simulink model "EvPowertrainController"  (R2019b)
settings: Solver=ode4  StartTime=0.0  StopTime=inf  FixedStep=.01  RelTol=1e-3  EnableMultiTasking=on
model workspace (MAT data in the model file):
  BattChrgMax = -80000
  BattDischrgMax = 80000
  BrkPrsMax = 5000000
  ChrgLmt_bpt = [1 1 1 1 1 1 1 1 0.7 0.35 0]
  DischrgLmt_bpt = [0 0.35 0.7 1 1 1 1 1 1 1 1]
  MotMapEff = 0
  MotSpd = [0 1000 2000 2728.370453 3000 4000 5000 6000 7000 8000 9000 10000]
  MotTrq = [280 280 280 280 254.6479089 190.9859317 152.7887454 127.3239545 109.1348181 95.49296586 84.88263632 76.39437268]
  Ndiff = 7.94
  RegenBrkCutOff = [0 1]
  RegenBrkSpd_bpt = [5 9]
  Rm = 0.15
  SOC_bpt = [0 10 20 30 40 50 60 70 80 90 100]
  T_eff_bp = [0 20 40 60 80 100 120 140 160 180 200 220 240 260 280]
  disk_abore = 0.05
  efficiency_table = [85  85  85  85  85  85  85  85  85  85  85  85  85  85  85; 85  85  85  85  85  85  85  85  85  85  85  85  85  85  85; 85  85  90  90  90  90  90  90  90  90  88  88  88  88  88; 85  85  92  92  92  92  92  92  92  92  92  90  90  90  90; 85  85  92  92  93  93  93  93  92  92  92  90  90  90  90; 85  85  93  94  94  94  94  94  94  94  94  94  94  94  94; 85  85  93  94  94  95  95  95  95  95  95  95  95  95  95; 85  85  93  94  94  95  95  95  95  95  95  95  95  95  95; 85  85  93  94  95  95  95  95  95  95  95  95  95  95  95; 85  85  93  94  95  95  95  95  95  95  95  95  95  95  95; 85  85  93  94  94  94  94  94  94  94  94  94  94  94  94; 85  85  90  92  93  93  93  93  93  93  93  93  93  93  93]
  mu_kinetic = 0.35
  num_pads = 2
  w_eff_bp = [0 1000 2000 2728.370453 3000 4000 5000 6000 7000 8000 9000 10000]
libraries: simulink x6, autolibutils x1
settings Model: ModifiedByFormat=The MathWorks, Inc.  Creator=The MathWorks, Inc.  LastModifiedBy=The MathWorks, Inc.
settings DataIOCC: ReturnWorkspaceOutputs=off
settings DebuggingCC: UnderspecifiedInitializationDetection=Classic  MergeDetectMultiDrivingBlocksExec=none  SFNoUnconditionalDefaultTransitionDiag=warning  ArithmeticOperatorsInVariantConditions=warning
settings SFSimCC: SimUseLocalCustomCode=off  CustomCodeUndefinedFunction=UseInterfaceOnly
settings RTWCC: RTWUseLocalCustomCode=off
settings CodeAppCC: StateflowObjectComments=on
settings GRTTargetCC: TargetLangStandard=C89/C90 (ANSI)
settings ConfigComp: CovMetricSettings=dsw  CovHtmlReporting=on  CovSaveCumulativeToWorkspaceVar=on  CovSaveSingleToWorkspaceVar=on  CovShowResultsExplorer=off  CovExternalEMLEnable=off

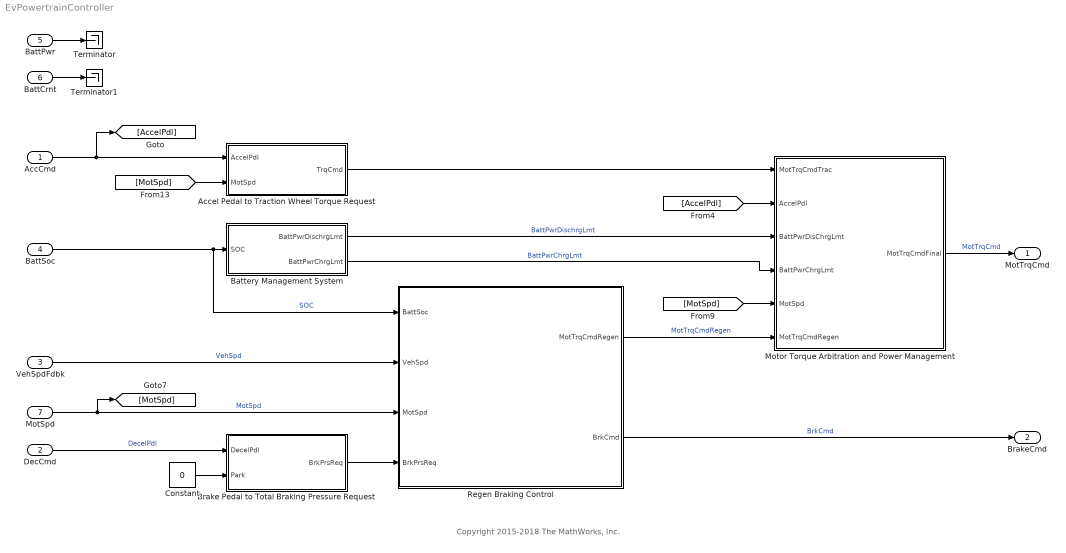
== system EvPowertrainController ==
  note: Copyright 2015-2018 The MathWorks, Inc.
  AccCmd : Inport
  DecCmd : Inport  Port=2  OutDataTypeStr=double
  VehSpdFdbk : Inport  Port=3
  BattSoc : Inport  Port=4
  BattPwr : Inport  Port=5
  BattCrnt : Inport  Port=6
  MotSpd : Inport  Port=7
  Accel Pedal to Traction Wheel Torque Request : Subsystem
  Battery Management System : Subsystem
  Brake Pedal to Total Braking Pressure Request : Subsystem
  Constant : Constant  Value=0
  Motor Torque Arbitration and Power Management : Subsystem
  Regen Braking Control : Subsystem  VariantControlMode=Label  Variant=on  VariantControl=(default)  LabelModeActiveChoice=Variant
  Terminator : Terminator
  Terminator1 : Terminator
  MotTrqCmd : Outport  VectorParamsAs1DForOutWhenUnconnected=off
  BrakeCmd : Outport  Port=2  VectorParamsAs1DForOutWhenUnconnected=off
  wires:
  [AccelPdl] -> Motor Torque Arbitration and Power Management/2(AccelPdl)
  Battery Management System/1(BattPwrDischrgLmt) -> Motor Torque Arbitration and Power Management/3(BattPwrDisChrgLmt)  "BattPwrDischrgLmt"
  DecCmd/1 -> Brake Pedal to Total Braking Pressure Request/1(DecelPdl)  "DecelPdl"
  Regen Braking Control/2(" BrkCmd") -> BrakeCmd/1  "BrkCmd"
  Constant/1 -> Brake Pedal to Total Braking Pressure Request/2(Park)
  Battery Management System/2(BattPwrChrgLmt) -> Motor Torque Arbitration and Power Management/4("BattPwrChrgLmt ")  "BattPwrChrgLmt"
  Brake Pedal to Total Braking Pressure Request/1(BrkPrsReq) -> Regen Braking Control/4("BrkPrsReq ")
  [MotSpd] -> Accel Pedal to Traction Wheel Torque Request/2(MotSpd)
  VehSpdFdbk/1 -> Regen Braking Control/2("VehSpd ")  "VehSpd"
  BattSoc/1 -> Regen Braking Control/1("BattSoc "), Battery Management System/1(SOC)  "SOC"
  Accel Pedal to Traction Wheel Torque Request/1(TrqCmd) -> Motor Torque Arbitration and Power Management/1(MotTrqCmdTrac)
  MotSpd/1 -> Regen Braking Control/3("MotSpd "), [MotSpd]  "MotSpd"
  AccCmd/1 -> [AccelPdl], Accel Pedal to Traction Wheel Torque Request/1(AccelPdl)
  [MotSpd] -> Motor Torque Arbitration and Power Management/5(MotSpd)
  Motor Torque Arbitration and Power Management/1(MotTrqCmdFinal) -> MotTrqCmd/1  "MotTrqCmd"
  Regen Braking Control/1(" MotTrqCmdRegen") -> Motor Torque Arbitration and Power Management/6(MotTrqCmdRegen)  "MotTrqCmdRegen"
  BattPwr/1 -> Terminator/1
  BattCrnt/1 -> Terminator1/1

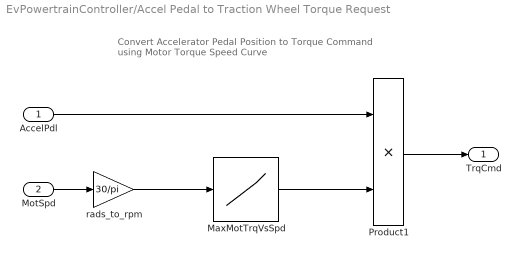
== system EvPowertrainController/Accel Pedal to Traction Wheel Torque Request ==
  note: Convert Accelerator Pedal Position to Torque Command
      | using Motor Torque Speed Curve
  AccelPdl : Inport
  MotSpd : Inport  Port=2
  MaxMotTrqVsSpd : Lookup_n-D  NumberOfTableDimensions=1  BreakpointsForDimension1=MotSpd  Table=MotTrq  ExtrapMethod=Clip  UseLastTableValue=on  InternalRulePriority=Speed  OutDataTypeStr=Inherit: Inherit from 'Table data'  RndMeth=Simplest  InputSameDT=on
  Product1 : Product
  rads_to_rpm : Gain  Gain=30/pi
  TrqCmd : Outport  VectorParamsAs1DForOutWhenUnconnected=off
  wires:
  Product1/1 -> TrqCmd/1
  MaxMotTrqVsSpd/1 -> Product1/2
  AccelPdl/1 -> Product1/1
  MotSpd/1 -> rads_to_rpm/1
  rads_to_rpm/1 -> MaxMotTrqVsSpd/1

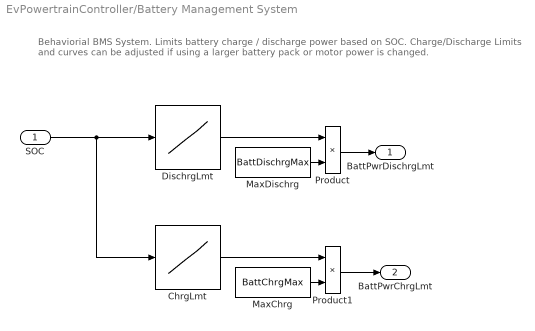
== system EvPowertrainController/Battery Management System ==
  note: Behaviorial BMS System. Limits battery charge / discharge power based on SOC.
      |
      | Charge/Discharge Limits and curves can be adjusted if using a larger battery pack
      | or motor power is changed.
  SOC : Inport
  ChrgLmt : Lookup_n-D  NumberOfTableDimensions=1  BreakpointsForDimension1=SOC_bpt  Table=ChrgLmt_bpt  ExtrapMethod=Clip  UseLastTableValue=on  InternalRulePriority=Speed  RndMeth=Simplest  InputSameDT=on
  DischrgLmt : Lookup_n-D  NumberOfTableDimensions=1  BreakpointsForDimension1=SOC_bpt  Table=DischrgLmt_bpt  ExtrapMethod=Clip  UseLastTableValue=on  InternalRulePriority=Speed  RndMeth=Simplest  InputSameDT=on
  MaxChrg : Constant  Value=BattChrgMax
  MaxDischrg : Constant  Value=BattDischrgMax
  Product : Product
  Product1 : Product
  BattPwrDischrgLmt : Outport  VectorParamsAs1DForOutWhenUnconnected=off
  BattPwrChrgLmt : Outport  Port=2  VectorParamsAs1DForOutWhenUnconnected=off
  wires:
  SOC/1 -> DischrgLmt/1, ChrgLmt/1
  MaxChrg/1 -> Product1/2
  MaxDischrg/1 -> Product/2
  Product/1 -> BattPwrDischrgLmt/1
  Product1/1 -> BattPwrChrgLmt/1
  ChrgLmt/1 -> Product1/1
  DischrgLmt/1 -> Product/1

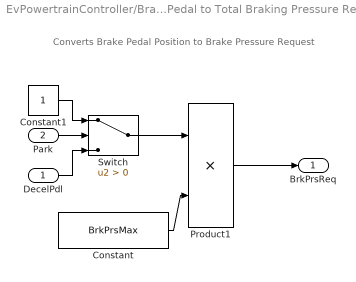
== system EvPowertrainController/Brake Pedal to Total Braking Pressure Request ==
  note: Converts Brake Pedal Position to Brake Pressure Request
  DecelPdl : Inport
  Park : Inport  Port=2
  Constant : Constant  Value=BrkPrsMax
  Constant1 : Constant
  Product1 : Product
  Switch : Switch  Criteria=u2 > Threshold
  BrkPrsReq : Outport  VectorParamsAs1DForOutWhenUnconnected=off
  wires:
  Constant/1 -> Product1/2
  Switch/1 -> Product1/1
  DecelPdl/1 -> Switch/3
  Constant1/1 -> Switch/1
  Product1/1 -> BrkPrsReq/1
  Park/1 -> Switch/2

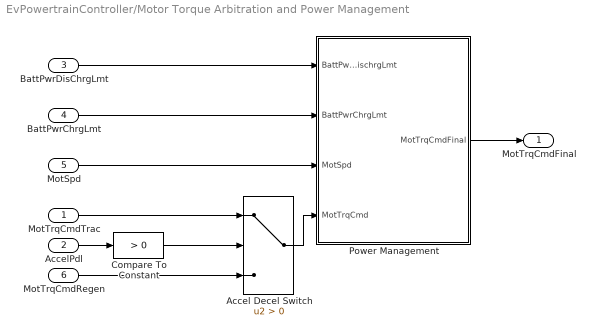
== system EvPowertrainController/Motor Torque Arbitration and Power Management ==
  MotTrqCmdTrac : Inport
  AccelPdl : Inport  Port=2
  BattPwrDisChrgLmt : Inport  Port=3
  "BattPwrChrgLmt " : Inport  Port=4
  MotSpd : Inport  Port=5
  MotTrqCmdRegen : Inport  Port=6
  Accel Decel Switch : Switch  Criteria=u2 > Threshold
  Compare To Constant : simulink/Logic and Bit Operations/Compare To Constant  relop=>  const=0  OutDataTypeStr=boolean
  Power Management : Subsystem
  MotTrqCmdFinal : Outport  VectorParamsAs1DForOutWhenUnconnected=off
  wires:
  AccelPdl/1 -> Compare To Constant/1
  MotTrqCmdRegen/1 -> Accel Decel Switch/3
  MotTrqCmdTrac/1 -> Accel Decel Switch/1
  Power Management/1(MotTrqCmdFinal) -> MotTrqCmdFinal/1
  Accel Decel Switch/1 -> Power Management/4(MotTrqCmd)
  BattPwrDisChrgLmt/1 -> Power Management/1(BattPwrDischrgLmt)
  "BattPwrChrgLmt "/1 -> Power Management/2(BattPwrChrgLmt)
  MotSpd/1 -> Power Management/3(MotSpd)
  Compare To Constant/1 -> Accel Decel Switch/2

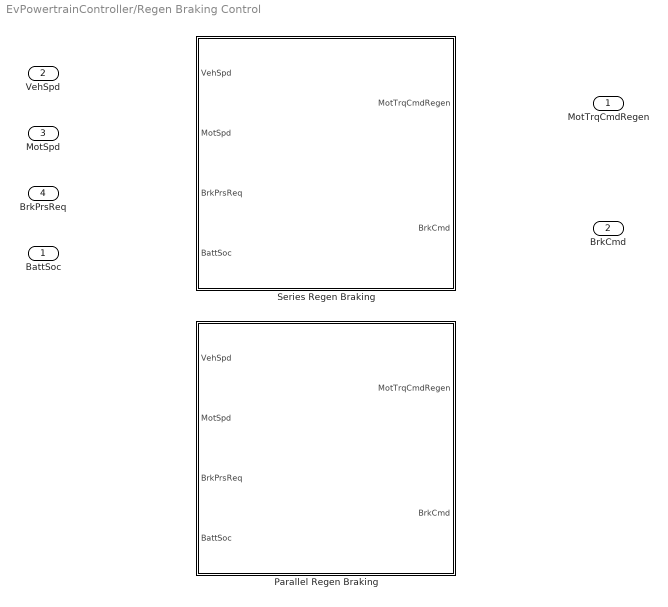
== system EvPowertrainController/Regen Braking Control ==
  "BattSoc " : Inport
  "VehSpd " : Inport  Port=2
  "MotSpd " : Inport  Port=3
  "BrkPrsReq " : Inport  Port=4
  Parallel Regen Braking : Subsystem  InitFcn=%[~]=autosharedicon('autolibutils',gcb,0);  VariantControl=(default)
  Series Regen Braking : Subsystem  InitFcn=%[~]=autosharedicon('autolibutils',gcb,0);  VariantControl=Variant
  " MotTrqCmdRegen" : Outport  VectorParamsAs1DForOutWhenUnconnected=off
  " BrkCmd" : Outport  Port=2  VectorParamsAs1DForOutWhenUnconnected=off

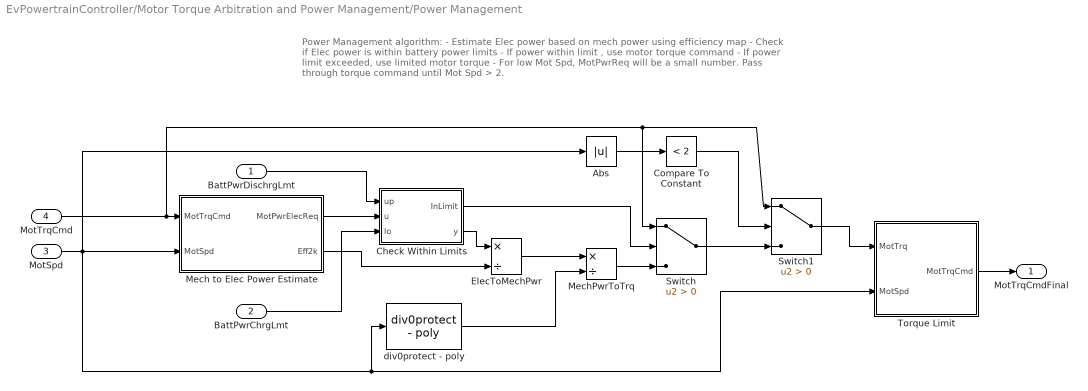
== system EvPowertrainController/Motor Torque Arbitration and Power Management/Power Management ==
  note: Power Management algorithm:
      | - Estimate Elec power based on mech power using efficiency map
      | - Check if Elec power is within battery power limits
      | - If power within limit , use motor torque command
      | - If power limit exceeded, use limited motor torque
      | - For low Mot Spd, MotPwrReq will be a small number.  Pass through torque command until Mot Spd > 2.
  BattPwrDischrgLmt : Inport
  BattPwrChrgLmt : Inport  Port=2
  MotSpd : Inport  Port=3
  MotTrqCmd : Inport  Port=4
  Abs : Abs
  Check Within Limits : Subsystem
  Compare To Constant : simulink/Logic and Bit Operations/Compare To Constant  relop=<  const=2  OutDataTypeStr=boolean
  ElecToMechPwr : Product  Inputs=*/
  Mech to Elec Power Estimate : Subsystem
  MechPwrToTrq : Product  Inputs=*/
  Switch : Switch  Criteria=u2 > Threshold
  Switch1 : Switch  Criteria=u2 > Threshold
  Torque Limit : Subsystem
  div0protect - poly : autolibutils/div0protect - poly  thresh=2  aMode=aMode
      settings: SourceProductName=Powertrain Blockset  SourceProductBaseCode=PW
  MotTrqCmdFinal : Outport  VectorParamsAs1DForOutWhenUnconnected=off
  wires:
  MotSpd/1 -> Abs/1, Torque Limit/2(MotSpd), div0protect - poly/1, Mech to Elec Power Estimate/2(MotSpd)
  MotTrqCmd/1 -> Switch/1, Switch1/1, Mech to Elec Power Estimate/1(MotTrqCmd)
  div0protect - poly/1 -> MechPwrToTrq/2
  Mech to Elec Power Estimate/2(Eff2k) -> ElecToMechPwr/2
  ElecToMechPwr/1 -> MechPwrToTrq/1
  MechPwrToTrq/1 -> Switch/3
  Torque Limit/1(MotTrqCmd) -> MotTrqCmdFinal/1
  BattPwrDischrgLmt/1 -> Check Within Limits/1(up)
  Mech to Elec Power Estimate/1(MotPwrElecReq) -> Check Within Limits/2(u)
  BattPwrChrgLmt/1 -> Check Within Limits/3(lo)
  Check Within Limits/2(y) -> ElecToMechPwr/1
  Switch/1 -> Switch1/3
  Check Within Limits/1(InLimit) -> Switch/2
  Switch1/1 -> Torque Limit/1(MotTrq)
  Abs/1 -> Compare To Constant/1
  Compare To Constant/1 -> Switch1/2

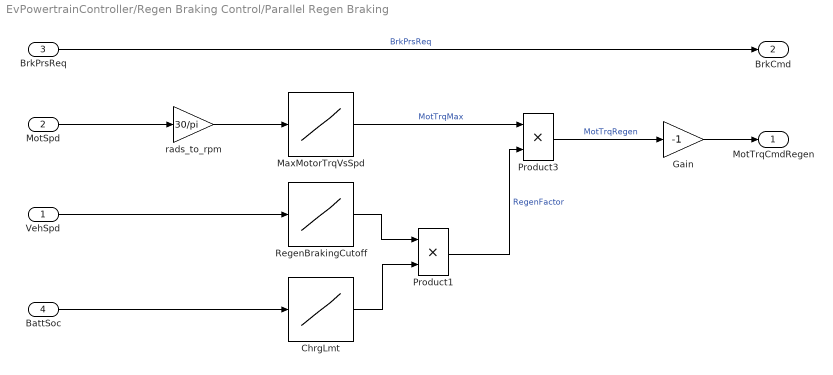
== system EvPowertrainController/Regen Braking Control/Parallel Regen Braking ==
  VehSpd : Inport
  MotSpd : Inport  Port=2
  "BrkPrsReq " : Inport  Port=3
  BattSoc : Inport  Port=4
  ChrgLmt : Lookup_n-D  NumberOfTableDimensions=1  BreakpointsForDimension1=[0:10:100]  Table=[1 1 1 1 1 1 1 1 0.7 0.35 0]  ExtrapMethod=Clip  UseLastTableValue=on  InternalRulePriority=Speed  RndMeth=Simplest  InputSameDT=on
  Gain : Gain  Gain=-1
  MaxMotorTrqVsSpd : Lookup_n-D  NumberOfTableDimensions=1  BreakpointsForDimension1=MotSpd  Table=MotTrq  ExtrapMethod=Clip  UseLastTableValue=on  InternalRulePriority=Speed  OutDataTypeStr=Inherit: Inherit from 'Table data'  RndMeth=Simplest  InputSameDT=on
  Product1 : Product
  Product3 : Product
  RegenBrakingCutoff : Lookup_n-D  NumberOfTableDimensions=1  BreakpointsForDimension1=[2.2 4.5]  Table=[0 1]  ExtrapMethod=Clip  UseLastTableValue=on  InternalRulePriority=Speed  RndMeth=Simplest  InputSameDT=on
  rads_to_rpm : Gain  Gain=30/pi
  " MotTrqCmdRegen" : Outport  VectorParamsAs1DForOutWhenUnconnected=off
  " BrkCmd" : Outport  Port=2  VectorParamsAs1DForOutWhenUnconnected=off
  wires:
  Gain/1 -> " MotTrqCmdRegen"/1
  BattSoc/1 -> ChrgLmt/1
  Product3/1 -> Gain/1  "MotTrqRegen"
  Product1/1 -> Product3/2  "RegenFactor"
  RegenBrakingCutoff/1 -> Product1/1
  VehSpd/1 -> RegenBrakingCutoff/1
  ChrgLmt/1 -> Product1/2
  MaxMotorTrqVsSpd/1 -> Product3/1  "MotTrqMax"
  rads_to_rpm/1 -> MaxMotorTrqVsSpd/1
  MotSpd/1 -> rads_to_rpm/1
  "BrkPrsReq "/1 -> " BrkCmd"/1  "BrkPrsReq"

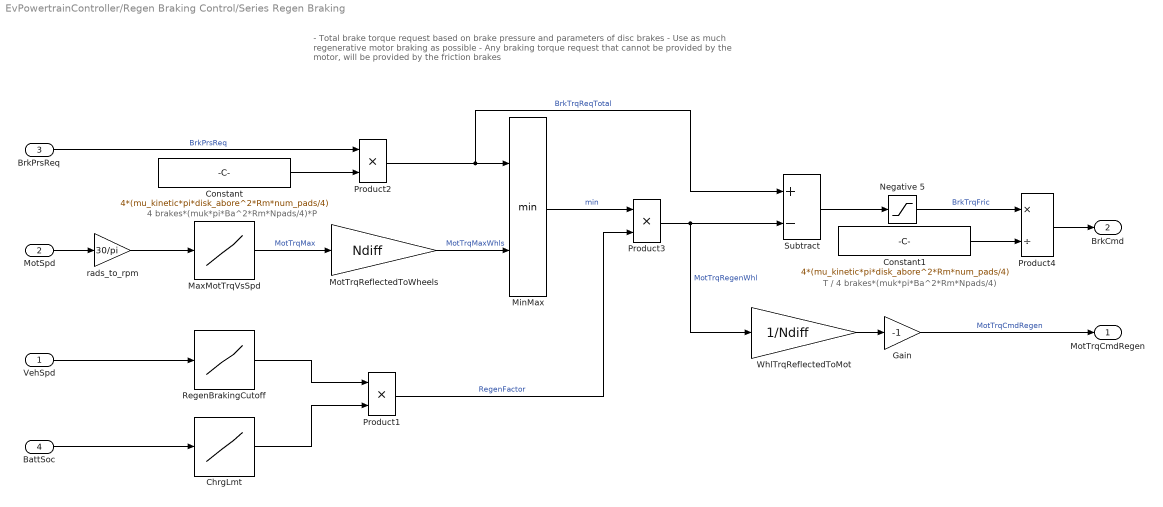
== system EvPowertrainController/Regen Braking Control/Series Regen Braking ==
  note: - Total brake torque request based on brake pressure and parameters of disc brakes
      | - Use as much regenerative motor braking as possible
      | - Any braking torque request that cannot be provided by the motor, will be provided by the friction brakes
  note: T / 4 brakes*(muk*pi*Ba^2*Rm*Npads/4)
  note: 4 brakes*(muk*pi*Ba^2*Rm*Npads/4)*P
  VehSpd : Inport
  MotSpd : Inport  Port=2
  "BrkPrsReq " : Inport  Port=3
  BattSoc : Inport  Port=4
  ChrgLmt : Lookup_n-D  NumberOfTableDimensions=1  BreakpointsForDimension1=SOC_bpt  Table=ChrgLmt_bpt  ExtrapMethod=Clip  UseLastTableValue=on  InternalRulePriority=Speed  RndMeth=Simplest  InputSameDT=on
  Constant : Constant  Value=4*(mu_kinetic*pi*disk_abore^2*Rm*num_pads/4)
  Constant1 : Constant  Value=4*(mu_kinetic*pi*disk_abore^2*Rm*num_pads/4)
  Gain : Gain  Gain=-1
  MaxMotTrqVsSpd : Lookup_n-D  NumberOfTableDimensions=1  BreakpointsForDimension1=MotSpd  Table=MotTrq  ExtrapMethod=Clip  UseLastTableValue=on  InternalRulePriority=Speed  OutDataTypeStr=Inherit: Inherit from 'Table data'  RndMeth=Simplest  InputSameDT=on
  MinMax : MinMax  Inputs=2
  MotTrqReflectedToWheels : Gain  Gain=Ndiff
  Negative 5 : Saturate  UpperLimit=inf  LowerLimit=0
  Product1 : Product
  Product2 : Product
  Product3 : Product
  Product4 : Product  Inputs=*/
  RegenBrakingCutoff : Lookup_n-D  NumberOfTableDimensions=1  BreakpointsForDimension1=RegenBrkSpd_bpt  Table=RegenBrkCutOff  ExtrapMethod=Clip  UseLastTableValue=on  InternalRulePriority=Speed  RndMeth=Simplest  InputSameDT=on
  Subtract : Sum  Inputs=+-
  WhlTrqReflectedToMot : Gain  Gain=1/Ndiff
  rads_to_rpm : Gain  Gain=30/pi
  " MotTrqCmdRegen" : Outport  VectorParamsAs1DForOutWhenUnconnected=off
  " BrkCmd" : Outport  Port=2  VectorParamsAs1DForOutWhenUnconnected=off
  wires:
  Product3/1 -> WhlTrqReflectedToMot/1, Subtract/2  "MotTrqRegenWhl"
  Product4/1 -> " BrkCmd"/1
  Constant1/1 -> Product4/2
  Constant/1 -> Product2/2
  "BrkPrsReq "/1 -> Product2/1  "BrkPrsReq"
  rads_to_rpm/1 -> MaxMotTrqVsSpd/1
  MaxMotTrqVsSpd/1 -> MotTrqReflectedToWheels/1  "MotTrqMax"
  Product2/1 -> MinMax/1, Subtract/1  "BrkTrqReqTotal"
  MinMax/1 -> Product3/1  "min"
  ChrgLmt/1 -> Product1/2
  VehSpd/1 -> RegenBrakingCutoff/1
  RegenBrakingCutoff/1 -> Product1/1
  Product1/1 -> Product3/2  "RegenFactor"
  Subtract/1 -> Negative 5/1
  BattSoc/1 -> ChrgLmt/1
  Negative 5/1 -> Product4/1  "BrkTrqFric"
  MotSpd/1 -> rads_to_rpm/1
  MotTrqReflectedToWheels/1 -> MinMax/2  "MotTrqMaxWhls"
  WhlTrqReflectedToMot/1 -> Gain/1
  Gain/1 -> " MotTrqCmdRegen"/1  "MotTrqCmdRegen"

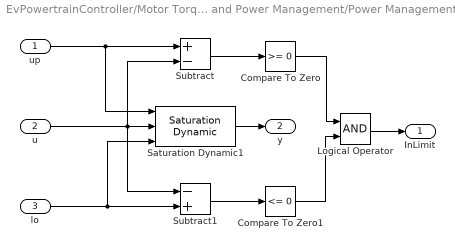
== system EvPowertrainController/Motor Torque Arbitration and Power Management/Power Management/Check Within Limits ==
  up : Inport
  u : Inport  Port=2
  lo : Inport  Port=3
  Compare To Zero : simulink/Logic and Bit Operations/Compare To Zero  relop=>=  OutDataTypeStr=boolean
  Compare To Zero1 : simulink/Logic and Bit Operations/Compare To Zero  relop=<=  OutDataTypeStr=boolean
  Logical Operator : Logic  AllPortsSameDT=off  OutDataTypeStr=boolean
  Saturation Dynamic1 : simulink/Discontinuities/Saturation Dynamic  OutMin=[]  OutMax=[]  OutDataTypeStr=Inherit: Same as second input  OutDataType=fixdt(1, 16)  OutScaling=2^-10  DoSatur=off
  Subtract : Sum  Inputs=+-
  Subtract1 : Sum  Inputs=-+
  InLimit : Outport  VectorParamsAs1DForOutWhenUnconnected=off
  y : Outport  Port=2  VectorParamsAs1DForOutWhenUnconnected=off
  wires:
  Saturation Dynamic1/1 -> y/1
  lo/1 -> Subtract1/2, Saturation Dynamic1/3
  up/1 -> Subtract/1, Saturation Dynamic1/1
  u/1 -> Subtract1/1, Subtract/2, Saturation Dynamic1/2
  Subtract/1 -> Compare To Zero/1
  Subtract1/1 -> Compare To Zero1/1
  Compare To Zero/1 -> Logical Operator/1
  Compare To Zero1/1 -> Logical Operator/2
  Logical Operator/1 -> InLimit/1

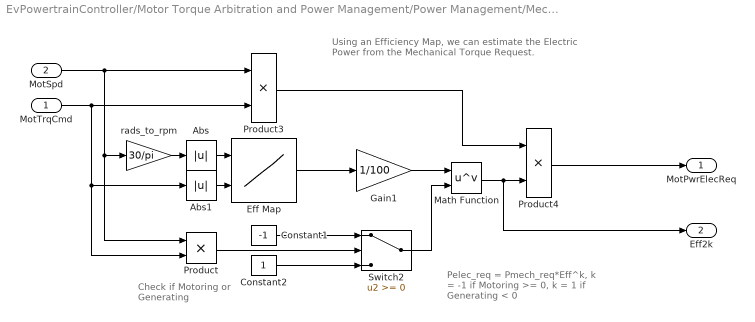
== system EvPowertrainController/Motor Torque Arbitration and Power Management/Power Management/Mech to Elec Power Estimate ==
  note: Check if Motoring
      | or Generating
  note: Using an Efficiency Map, we can estimate the
      | Electric Power from the Mechanical  Torque Request.
  note: Pelec_req = Pmech_req*Eff^k,
      | k = -1 if Motoring >= 0,
      | k = 1 if Generating < 0
  MotTrqCmd : Inport
  MotSpd : Inport  Port=2
  Abs : Abs
  Abs1 : Abs
  Constant1 : Constant  Value=-1  SampleTime=-1
  Constant2 : Constant  SampleTime=-1
  Eff Map : Lookup_n-D  BreakpointsForDimension1=w_eff_bp  BreakpointsForDimension2=T_eff_bp  Table=efficiency_table  ExtrapMethod=Clip  UseLastTableValue=on  InternalRulePriority=Speed  OutDataTypeStr=Inherit: Inherit from 'Table data'  RndMeth=Simplest  InputSameDT=on
  Gain1 : Gain  Gain=1/100
  Math Function : Math  Operator=pow  OutputSignalType=real  SaturateOnIntegerOverflow=on
  Product : Product
  Product3 : Product
  Product4 : Product
  Switch2 : Switch
  rads_to_rpm : Gain  Gain=30/pi
  MotPwrElecReq : Outport  VectorParamsAs1DForOutWhenUnconnected=off
  Eff2k : Outport  Port=2  VectorParamsAs1DForOutWhenUnconnected=off
  wires:
  Product3/1 -> Product4/1
  Switch2/1 -> Math Function/2
  Constant1/1 -> Switch2/1
  Constant2/1 -> Switch2/3
  Eff Map/1 -> Gain1/1
  Abs/1 -> Eff Map/1
  Gain1/1 -> Math Function/1
  Math Function/1 -> Eff2k/1, Product4/2
  Product4/1 -> MotPwrElecReq/1
  Abs1/1 -> Eff Map/2
  rads_to_rpm/1 -> Abs/1
  Product/1 -> Switch2/2
  MotSpd/1 -> Product3/1, Product/1, rads_to_rpm/1
  MotTrqCmd/1 -> Product3/2, Product/2, Abs1/1

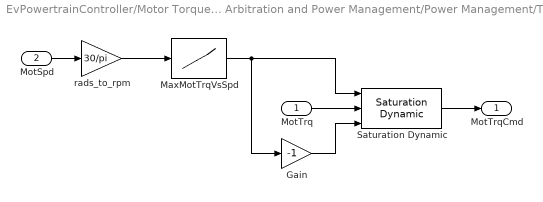
== system EvPowertrainController/Motor Torque Arbitration and Power Management/Power Management/Torque Limit ==
  MotTrq : Inport
  MotSpd : Inport  Port=2
  Gain : Gain  Gain=-1
  MaxMotTrqVsSpd : Lookup_n-D  NumberOfTableDimensions=1  BreakpointsForDimension1=MotSpd  Table=MotTrq  ExtrapMethod=Clip  UseLastTableValue=on  InternalRulePriority=Speed  OutDataTypeStr=Inherit: Inherit from 'Table data'  RndMeth=Simplest  InputSameDT=on
  Saturation Dynamic : simulink/Discontinuities/Saturation Dynamic  OutMin=[]  OutMax=[]  OutDataTypeStr=Inherit: Same as second input  OutDataType=fixdt(1, 16)  OutScaling=2^-10  DoSatur=off
  rads_to_rpm : Gain  Gain=30/pi
  MotTrqCmd : Outport  VectorParamsAs1DForOutWhenUnconnected=off
  wires:
  MotTrq/1 -> Saturation Dynamic/2
  Saturation Dynamic/1 -> MotTrqCmd/1
  MotSpd/1 -> rads_to_rpm/1
  MaxMotTrqVsSpd/1 -> Gain/1, Saturation Dynamic/1
  rads_to_rpm/1 -> MaxMotTrqVsSpd/1
  Gain/1 -> Saturation Dynamic/3
